simulink model "gm_sampleModel1798_1_sub"  (R2023a)
settings: Solver=VariableStepAuto  StartTime=0.0  StopTime=10.0  RelTol=1e-3
libraries: simulink x2, hdlsllib x1
settings Model: Creator=user1  LastModifiedBy=user1
settings OptimizationCC: BlockReduction=off  ConditionallyExecuteInputs=off
settings DebuggingCC: InheritedTsInSrcMsg=none

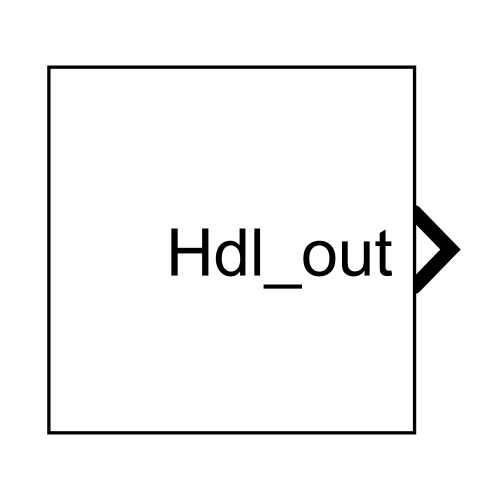
[thumbnail: Simulink's stored preview of the top-level diagram]
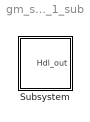
== system gm_sampleModel1798_1_sub ==
  Subsystem : Subsystem

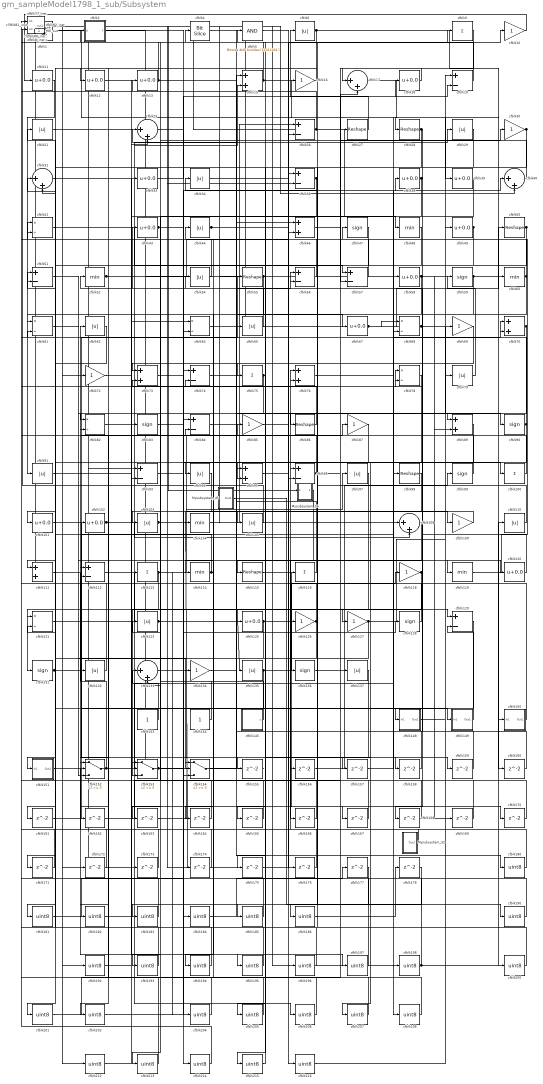
== system gm_sampleModel1798_1_sub/Subsystem ==
  Mysubsystem_32 : Subsystem
  Mysubsystem_36 : Subsystem
  Mysubsystem_45 : Subsystem
  cfblk1 : simulink/Logic and Bit Operations/Extract Bits  bitsToExtract=Upper half  numBits=8  bitIdxRange=[0 7]  outScalingMode=Preserve fixed-point scaling
      settings: LibrarySourceBlock=|
      | hdlsllib/Logic and Bit
      | Operations/Extract Bits
  cfblk{10,16,30,69,72,85,87,109,118,126..127,134} (12 alike) : Gain  OutDataTypeStr=uint8
  cfblk{9,75,100,113,116} (5 alike) : Sum  Inputs=+  OutDataTypeStr=uint8
  cfblk{11..13,18,33,38..39,43,49,58,67,101..102,120,125} (15 alike) : Bias  Bias=0.0  SaturateOnIntegerOverflow=off
  cfblk{6,21,29,34,44,54,62,65,79,91,94,97,103,105,110,123,132,135,137} (19 alike) : Abs  OutDataTypeStr=uint8  SaturateOnIntegerOverflow=off
  cfblk{48,52,60,104,114,119} (6 alike) : MinMax  OutDataTypeStr=uint8
  cfblk106_inst : Subsystem
  cfblk{17,23,31,40,108,133} (6 alike) : Sum  Inputs=|++  OutDataTypeStr=uint8
  cfblk{15,46,70,73,76,89,95,111} (8 alike) : Sum  OutDataTypeStr=uint8
  cfblk{19,26,36,51,56..57,74,84,93,96,112,129} (12 alike) : Sum  Inputs=+-  OutDataTypeStr=uint8
  cfblk{27..28,50,55,86,98,115} (7 alike) : Reshape
  cfblk117_inst : Subsystem
  cfblk{41,61,64,68,78,82,121} (7 alike) : Product  Inputs=*/  OutDataTypeStr=uint8  RndMeth=Zero  SaturateOnIntegerOverflow=on
  cfblk122_inst : Subsystem
  cfblk{47,59,83,90,99,128,131,136} (8 alike) : Signum
  cfblk130_inst : Subsystem
  cfblk143 : Constant  OutDataTypeStr=uint8  SampleTime=-1
  cfblk144 : Constant  OutDataTypeStr=uint8  SampleTime=-1
  cfblk145 : Subsystem  mask(Counter Limited){uplimit=double(7), tsamp=double(-1)}
      mask prompts: uplimit "Simulink:masks:UpperLimit_MP"; tsamp "Simulink:masks:SampleTime_MP"
      mask help: Simulink:masks:CounterLimited_MD
      mask init:
      | nbits = double(8);
      | tsamp = double(-1);
      | uplimit = double(7);
  cfblk148 : Subsystem
  cfblk149 : Subsystem
  cfblk150 : Subsystem
  cfblk151 : Subsystem
  cfblk152 : Switch  OutDataTypeStr=uint8  SaturateOnIntegerOverflow=off  InputSameDT=off
  cfblk153 : Switch  OutDataTypeStr=uint8  SaturateOnIntegerOverflow=off  InputSameDT=off
  cfblk154 : Switch  OutDataTypeStr=uint8  SaturateOnIntegerOverflow=off  InputSameDT=off
  cfblk{155..178} (24 alike) : Delay  SampleTime=1
  cfblk{180..186,190,192..198,200..202,204..208,212..216} (28 alike) : DataTypeConversion  OutDataTypeStr=uint8  SaturateOnIntegerOverflow=off  RndMeth=Floor
  cfblk2 : Subsystem  mask(Detect Rise Positive){vinit=double(0), InputProcessing=Elements as channels (sample based), OutDataTypeStr=uint8}
      mask prompts: vinit "Simulink:masks:InitialCondition_MP"; InputProcessing "Simulink:masks:InputProcessing_MP"; OutDataTypeStr "Simulink:masks:OutputDataType_MP"
      mask help: Simulink:masks:DetectRisePositive_MD
      mask init:
      | InputProcessing = 'Elements as channels (sample based)';
      | OutDataTypeStr = 'uint8';
      | vinit = double(0);
      mask TypeOptions InputProcessing: Simulink:masks:ColumnsAsChannelsFrameBased | Simulink:masks:ElementsAsChannelsSampleBased
      mask TypeOptions OutDataTypeStr: Simulink:masks:uint8 | Simulink:masks:boolean
      mask Display: fprintf('U > 0\n&  NOT\nU/z > 0')
  cfblk20_inst : Subsystem
  cfblk32_inst : Subsystem
  cfblk35_inst : Subsystem
  cfblk4 : hdlsllib/Logic and Bit Operations/Bit Slice  lidx=7  ridx=0
  cfblk45_inst : Subsystem
  cfblk5 : simulink/Logic and Bit Operations/Bitwise Operator  logicop=AND  UseBitMask=on  BitMask=bin2dec('11011001')  BitMaskRealWorld=Stored Integer
      settings: LibrarySourceBlock=|
      | hdlsllib/Logic and Bit
      | Operations/Bitwise
      | Operator
  cfblk53_inst : Subsystem
  cfblk63_inst : Subsystem
  cfblk77_inst : Subsystem
  cfblk80_inst : Subsystem
  cfblk81_inst : Subsystem
  cfblk8_inst : Subsystem
  cfblk92_inst : Subsystem
  Hdl_out : Outport  OutDataTypeStr=uint8  SampleTime=1
  wires:
  Mysubsystem_32/1(Out1) -> cfblk76/1
  Mysubsystem_36/1(Out1) -> cfblk166/1
  Mysubsystem_45/1(Out1) -> cfblk190/1
  cfblk1/1 -> cfblk28/1
  cfblk10/1 -> cfblk11/1
  cfblk100/1 -> cfblk34/1
  cfblk101/1 -> cfblk158/1
  cfblk102/1 -> cfblk29/1, cfblk108/2
  cfblk103/1 -> cfblk174/1, cfblk109/1
  cfblk104/1 -> cfblk26/1
  cfblk105/1 -> cfblk81_inst/2(in2)
  cfblk106_inst/1(out1) -> cfblk36/2, cfblk111/2
  cfblk108/1 -> cfblk115/1
  cfblk109/1 -> cfblk105/1
  cfblk11/1 -> cfblk91/1
  cfblk110/1 -> cfblk2/1(U)
  cfblk111/1 -> cfblk197/1
  cfblk112/1 -> cfblk206/1
  cfblk113/1 -> cfblk97/1, cfblk204/1, cfblk153/3, cfblk85/1
  cfblk114/1 -> cfblk51/1, cfblk194/1
  cfblk115/1 -> cfblk159/1
  cfblk116/1 -> cfblk23/1
  cfblk117_inst/1(out1) -> cfblk108/1, cfblk172/1
  cfblk118/1 -> cfblk207/1, cfblk131/1
  cfblk119/1 -> cfblk47/1
  cfblk12/1 -> cfblk23/2
  cfblk120/1 -> cfblk52/1
  cfblk121/1 -> cfblk15/2
  cfblk122_inst/1(out1) -> cfblk192/1
  cfblk123/1 -> cfblk213/1, cfblk135/1
  cfblk125/1 -> cfblk167/1, cfblk151/1(In1)
  cfblk126/1 -> cfblk96/1, cfblk154/2
  cfblk127/1 -> cfblk49/1, cfblk171/1
  cfblk128/1 -> cfblk62/1
  cfblk129/1 -> cfblk181/1
  cfblk13/1 -> cfblk77_inst/1(in1), cfblk119/1
  cfblk130_inst/1(out1) -> cfblk93/1, cfblk176/1
  cfblk131/1 -> cfblk84/2, cfblk149/1(In1)
  cfblk132/1 -> cfblk45_inst/2(in2)
  cfblk133/1 -> cfblk155/1
  cfblk134/1 -> cfblk46/1
  cfblk135/1 -> cfblk154/1, cfblk118/1
  cfblk136/1 -> cfblk99/1
  cfblk137/1 -> cfblk205/1
  cfblk143/1 -> cfblk133/1
  cfblk144/1 -> cfblk117_inst/2(in2)
  cfblk145/1(y) -> cfblk41/1
  cfblk148/1(Out1) -> cfblk70/1
  cfblk149/1(Out1) -> cfblk129/2
  cfblk15/1 -> cfblk4/1, cfblk68/2, cfblk150/1(In1)
  cfblk150/1(Out1) -> cfblk56/1
  cfblk151/1(Out1) -> cfblk55/1
  cfblk152/1 -> cfblk98/1, cfblk102/1
  cfblk153/1 -> cfblk128/1, cfblk123/1
  cfblk154/1 -> cfblk56/2
  cfblk155/1 -> cfblk1/1
  cfblk156/1 -> cfblk19/1
  cfblk157/1 -> cfblk40/1
  cfblk158/1 -> cfblk15/1
  cfblk159/1 -> cfblk78/1
  cfblk16/1 -> cfblk12/1
  cfblk160/1 -> cfblk36/1
  cfblk161/1 -> cfblk70/2
  cfblk162/1 -> cfblk46/2
  cfblk163/1 -> cfblk17/2
  cfblk164/1 -> cfblk63_inst/2(in2)
  cfblk165/1 -> cfblk32_inst/2(in2)
  cfblk166/1 -> cfblk61/2
  cfblk167/1 -> cfblk51/2
  cfblk168/1 -> cfblk121/2
  cfblk169/1 -> cfblk73/2
  cfblk17/1 -> cfblk39/1
  cfblk170/1 -> cfblk153/1
  cfblk171/1 -> cfblk130_inst/1(in1)
  cfblk172/1 -> cfblk81_inst/1(in1)
  cfblk173/1 -> cfblk82/2
  cfblk174/1 -> cfblk152/2
  cfblk175/1 -> cfblk26/2
  cfblk176/1 -> cfblk106_inst/2(in2)
  cfblk177/1 -> cfblk183/1
  cfblk178/1 -> cfblk185/1
  cfblk18/1 -> cfblk17/1
  cfblk180/1 -> cfblk35_inst/2(in2)
  cfblk181/1 -> cfblk74/1
  cfblk182/1 -> cfblk74/2
  cfblk183/1 -> cfblk35_inst/1(in1)
  cfblk184/1 -> cfblk177/1
  cfblk185/1 -> cfblk8_inst/1(in1)
  cfblk186/1 -> cfblk178/1
  cfblk19/1 -> cfblk106_inst/1(in1)
  cfblk190/1 -> cfblk8_inst/2(in2)
  cfblk192/1 -> cfblk33/1
  cfblk193/1 -> cfblk122_inst/1(in1)
  cfblk194/1 -> cfblk122_inst/2(in2)
  cfblk195/1 -> cfblk20_inst/2(in2)
  cfblk196/1 -> cfblk31/1
  cfblk197/1 -> cfblk31/2
  cfblk198/1 -> cfblk20_inst/1(in1), cfblk110/1
  cfblk2/1(Y) -> cfblk184/1
  cfblk20_inst/1(out1) -> cfblk58/1
  cfblk200/1 -> cfblk76/2
  cfblk201/1 -> cfblk137/1
  cfblk202/1 -> cfblk87/1
  cfblk204/1 -> cfblk80_inst/1(in1)
  cfblk205/1 -> cfblk80_inst/2(in2)
  cfblk206/1 -> cfblk44/1
  cfblk207/1 -> cfblk112/1
  cfblk208/1 -> cfblk112/2
  cfblk21/1 -> cfblk48/1
  cfblk212/1 -> cfblk64/1
  cfblk213/1 -> cfblk92_inst/1(in1)
  cfblk214/1 -> cfblk92_inst/2(in2)
  cfblk215/1 -> cfblk5/1
  cfblk216/1 -> cfblk79/1
  cfblk23/1 -> cfblk84/1
  cfblk26/1 -> cfblk208/1, cfblk130_inst/2(in2)
  cfblk27/1 -> cfblk6/1
  cfblk28/1 -> cfblk182/1, cfblk148/1(In1)
  cfblk29/1 -> cfblk101/1
  cfblk30/1 -> cfblk136/1, cfblk125/1
  cfblk31/1 -> cfblk195/1
  cfblk32_inst/1(out1) -> cfblk40/2
  cfblk33/1 -> cfblk18/1
  cfblk34/1 -> cfblk196/1
  cfblk35_inst/1(out1) -> cfblk200/1
  cfblk36/1 -> cfblk86/1, cfblk133/2
  cfblk38/1 -> cfblk95/2, cfblk75/1
  cfblk39/1 -> cfblk96/2
  cfblk4/1 -> cfblk67/1
  cfblk40/1 -> cfblk13/1
  cfblk41/1 -> cfblk57/1
  cfblk43/1 -> cfblk214/1, cfblk100/1
  cfblk44/1 -> cfblk65/1, cfblk10/1
  cfblk45_inst/1(out1) -> cfblk27/1
  cfblk46/1 -> cfblk19/2
  cfblk47/1 -> cfblk61/1
  cfblk48/1 -> cfblk64/2
  cfblk49/1 -> cfblk103/1, cfblk175/1
  cfblk5/1 -> cfblk216/1
  cfblk50/1 -> cfblk93/2, cfblk41/2
  cfblk51/1 -> cfblk134/1
  cfblk52/1 -> cfblk153/2, cfblk16/1
  cfblk53_inst/1(out1) -> cfblk60/1
  cfblk54/1 -> cfblk53_inst/1(in1)
  cfblk55/1 -> cfblk202/1, cfblk165/1, cfblk164/1, Hdl_out/1
  cfblk56/1 -> cfblk63_inst/1(in1)
  cfblk57/1 -> cfblk45_inst/1(in1)
  cfblk58/1 -> cfblk94/1, cfblk169/1, cfblk168/1
  cfblk59/1 -> cfblk152/1, cfblk111/1
  cfblk6/1 -> cfblk162/1, cfblk161/1, cfblk160/1
  cfblk60/1 -> cfblk21/1, cfblk132/1, cfblk163/1
  cfblk61/1 -> cfblk120/1
  cfblk62/1 -> cfblk121/1
  cfblk63_inst/1(out1) -> cfblk69/1
  cfblk64/1 -> cfblk89/1
  cfblk65/1 -> cfblk43/1
  cfblk67/1 -> cfblk50/1, cfblk68/1
  cfblk68/1 -> cfblk90/1, cfblk89/2
  cfblk69/1 -> cfblk73/1
  cfblk70/1 -> cfblk152/3, cfblk114/1
  cfblk72/1 -> cfblk126/1
  cfblk73/1 -> cfblk38/1
  cfblk74/1 -> cfblk180/1
  cfblk75/1 -> cfblk95/1, cfblk82/1
  cfblk76/1 -> cfblk198/1
  cfblk77_inst/1(out1) -> cfblk72/1
  cfblk78/1 -> cfblk215/1
  cfblk79/1 -> cfblk59/1
  cfblk8_inst/1(out1) -> cfblk113/1
  cfblk80_inst/1(out1) -> Mysubsystem_36/1(In1)
  cfblk81_inst/1(out1) -> cfblk117_inst/1(in1), cfblk173/1
  cfblk82/1 -> cfblk83/1
  cfblk83/1 -> cfblk78/2
  cfblk84/1 -> cfblk156/1
  cfblk85/1 -> cfblk9/1
  cfblk86/1 -> cfblk32_inst/1(in1)
  cfblk87/1 -> cfblk201/1
  cfblk89/1 -> cfblk116/1
  cfblk9/1 -> cfblk57/2
  cfblk90/1 -> cfblk77_inst/2(in2), cfblk154/3, cfblk157/1
  cfblk91/1 -> cfblk170/1
  cfblk92_inst/1(out1) -> cfblk212/1
  cfblk93/1 -> cfblk127/1
  cfblk94/1 -> cfblk193/1
  cfblk95/1 -> cfblk129/1
  cfblk96/1 -> cfblk53_inst/2(in2), cfblk30/1
  cfblk97/1 -> cfblk186/1
  cfblk98/1 -> cfblk104/1
  cfblk99/1 -> cfblk54/1

== system gm_sampleModel1798_1_sub/Subsystem/Mysubsystem_32 ==
  cfblk147 : Subsystem  mask(Counter Free-Running){NumBits=double(16), tsamp=double(-1)}
      mask prompts: NumBits "Simulink:masks:NumberOfBits_MP"; tsamp "Simulink:masks:SampleTime_MP"
      mask help: Simulink:masks:CounterFreeRunning_MD
  cfblk199 : DataTypeConversion  OutDataTypeStr=uint8  SaturateOnIntegerOverflow=off  RndMeth=Floor
  Out1 : Outport  SampleTime=1
  wires:
  cfblk147/1(y) -> cfblk199/1
  cfblk199/1 -> Out1/1

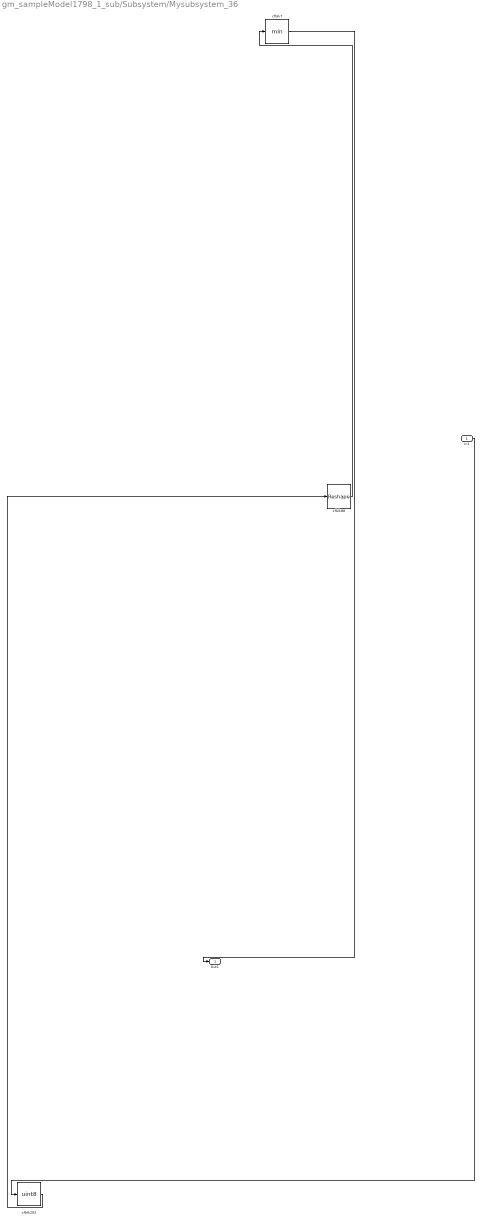
== system gm_sampleModel1798_1_sub/Subsystem/Mysubsystem_36 ==
  In1 : Inport  OutDataTypeStr=uint8  PortDimensions=1  SampleTime=1
  cfblk203 : DataTypeConversion  OutDataTypeStr=uint8  SaturateOnIntegerOverflow=off  RndMeth=Floor
  cfblk7 : MinMax
  cfblk88 : Reshape
  Out1 : Outport  SampleTime=1
  wires:
  In1/1 -> cfblk203/1
  cfblk203/1 -> cfblk88/1
  cfblk7/1 -> Out1/1
  cfblk88/1 -> cfblk7/1

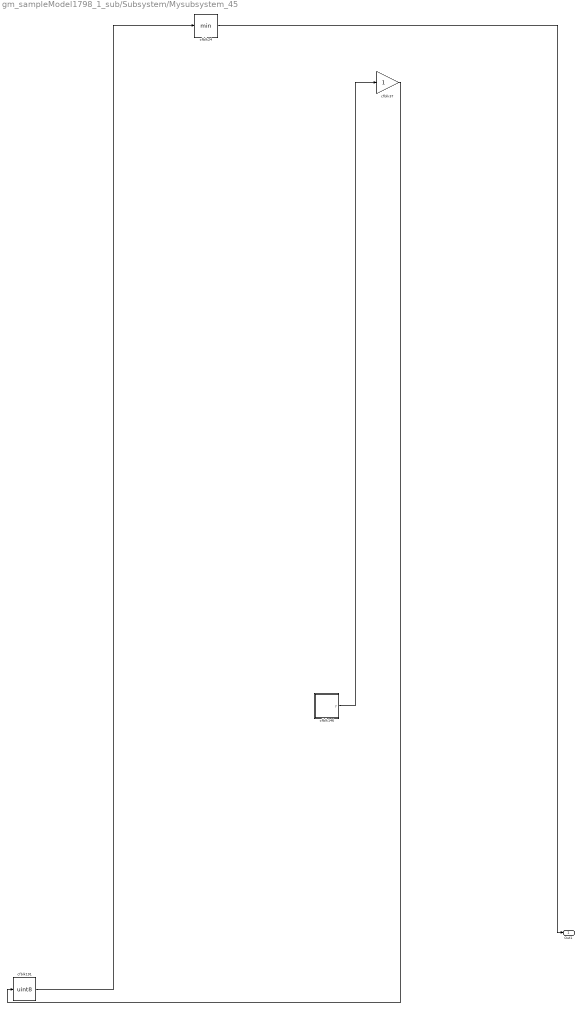
== system gm_sampleModel1798_1_sub/Subsystem/Mysubsystem_45 ==
  cfblk146 : Subsystem  mask(Counter Limited){uplimit=double(7), tsamp=double(-1)}
      mask prompts: uplimit "Simulink:masks:UpperLimit_MP"; tsamp "Simulink:masks:SampleTime_MP"
      mask help: Simulink:masks:CounterLimited_MD
      mask init:
      | nbits = double(8);
      | tsamp = double(-1);
      | uplimit = double(7);
  cfblk191 : DataTypeConversion  OutDataTypeStr=uint8  SaturateOnIntegerOverflow=off  RndMeth=Floor
  cfblk24 : MinMax
  cfblk37 : Gain
  Out1 : Outport  SampleTime=1
  wires:
  cfblk146/1(y) -> cfblk37/1
  cfblk191/1 -> cfblk24/1
  cfblk24/1 -> Out1/1
  cfblk37/1 -> cfblk191/1

== system gm_sampleModel1798_1_sub/Subsystem/cfblk106_inst ==
  in1 : Inport  OutDataTypeStr=uint8  SampleTime=1
  in2 : Inport  Port=2  OutDataTypeStr=uint8  SampleTime=1
  mul_cfblk106_dotp_mulcomp : Product  Inputs=**  OutDataTypeStr=uint8  SampleTime=1
  out1 : Outport  OutDataTypeStr=uint8  SampleTime=1
  wires:
  in1/1 -> mul_cfblk106_dotp_mulcomp/1
  in2/1 -> mul_cfblk106_dotp_mulcomp/2
  mul_cfblk106_dotp_mulcomp/1 -> out1/1

== system gm_sampleModel1798_1_sub/Subsystem/cfblk117_inst ==
  in1 : Inport  OutDataTypeStr=uint8  SampleTime=1
  in2 : Inport  Port=2  OutDataTypeStr=uint8  SampleTime=1
  mul_cfblk117_dotp_mulcomp : Product  Inputs=**  OutDataTypeStr=uint8  SampleTime=1
  out1 : Outport  OutDataTypeStr=uint8  SampleTime=1
  wires:
  in1/1 -> mul_cfblk117_dotp_mulcomp/1
  in2/1 -> mul_cfblk117_dotp_mulcomp/2
  mul_cfblk117_dotp_mulcomp/1 -> out1/1

== system gm_sampleModel1798_1_sub/Subsystem/cfblk122_inst ==
  in1 : Inport  OutDataTypeStr=uint8  SampleTime=1
  in2 : Inport  Port=2  OutDataTypeStr=uint8  SampleTime=1
  mul_cfblk122_dotp_mulcomp : Product  Inputs=**  OutDataTypeStr=uint8  SampleTime=1
  out1 : Outport  OutDataTypeStr=uint8  SampleTime=1
  wires:
  in1/1 -> mul_cfblk122_dotp_mulcomp/1
  in2/1 -> mul_cfblk122_dotp_mulcomp/2
  mul_cfblk122_dotp_mulcomp/1 -> out1/1

== system gm_sampleModel1798_1_sub/Subsystem/cfblk130_inst ==
  in1 : Inport  OutDataTypeStr=uint8  SampleTime=1
  in2 : Inport  Port=2  OutDataTypeStr=uint8  SampleTime=1
  mul_cfblk130_dotp_mulcomp : Product  Inputs=**  OutDataTypeStr=uint8  SampleTime=1
  out1 : Outport  OutDataTypeStr=uint8  SampleTime=1
  wires:
  in1/1 -> mul_cfblk130_dotp_mulcomp/1
  in2/1 -> mul_cfblk130_dotp_mulcomp/2
  mul_cfblk130_dotp_mulcomp/1 -> out1/1

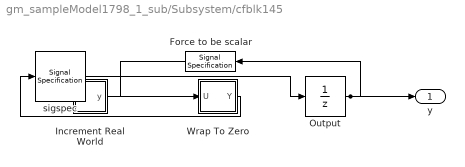
== system gm_sampleModel1798_1_sub/Subsystem/cfblk145 ==
  Force to be scalar : SignalSpecification  DisableCoverage=on  Dimensions=1
  Increment Real World : Subsystem  mask(Real World Value Increment){}
      mask help: Simulink:masks:RealWorldValueIncrement_MD
      mask Display: disp('V++')
  Output : UnitDelay  InitialCondition=0.0  SampleTime=tsamp  HasFrameUpgradeWarning=on
  Wrap To Zero : Subsystem  mask(Wrap To Zero){Threshold=double(7)}
      mask prompts: Threshold "Simulink:masks:Threshold_MP"
      mask help: Simulink:masks:WrapToZero_MD
  sigspec : SignalSpecification  OutDataTypeStr=uint8  Dimensions=1
  y : Outport  SampleTime=1
  wires:
  Force to be scalar/1 -> Increment Real World/1(u)
  Increment Real World/1(y) -> Wrap To Zero/1(U)
  Output/1 -> Force to be scalar/1, y/1
  Wrap To Zero/1(Y) -> sigspec/1
  sigspec/1 -> Output/1

== system gm_sampleModel1798_1_sub/Subsystem/cfblk148 ==
  In1 : Inport  OutDataTypeStr=fixdt(0, 4, -4)  PortDimensions=1  SampleTime=1
  Out1 : Outport  SampleTime=1
  wires:
  In1/1 -> Out1/1

== system gm_sampleModel1798_1_sub/Subsystem/cfblk149 ==
  In1 : Inport  OutDataTypeStr=uint8  PortDimensions=1  SampleTime=1
  Out1 : Outport  SampleTime=1
  wires:
  In1/1 -> Out1/1

== system gm_sampleModel1798_1_sub/Subsystem/cfblk150 ==
  In1 : Inport  OutDataTypeStr=uint8  PortDimensions=1  SampleTime=1
  Out1 : Outport  SampleTime=1
  wires:
  In1/1 -> Out1/1

== system gm_sampleModel1798_1_sub/Subsystem/cfblk151 ==
  In1 : Inport  OutDataTypeStr=uint8  PortDimensions=1  SampleTime=1
  Out1 : Outport  SampleTime=1
  wires:
  In1/1 -> Out1/1

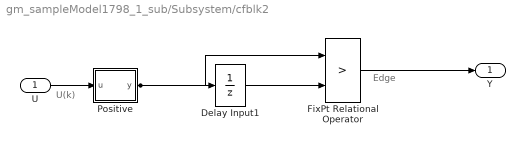
== system gm_sampleModel1798_1_sub/Subsystem/cfblk2 ==
  note: U(k)
  note: Edge
  U : Inport  OutDataTypeStr=uint8  SampleTime=1
  Delay Input1 : UnitDelay  Description=Store in Global RAM  DisableCoverage=on  InitialCondition=vinit  SampleTime=-1  HasFrameUpgradeWarning=on
  FixPt Relational Operator : RelationalOperator  Operator=>  OutDataTypeStr=fixdt(0, 8)  ZeroCross=off  InputSameDT=off
  Positive : Subsystem  mask(Compare To Zero){relop=>, OutDataTypeStr=boolean, ZeroCross=off}
      mask prompts: relop "Simulink:masks:Operator_MP"; OutDataTypeStr "Simulink:masks:OutputDataType_MP"; ZeroCross "Simulink:masks:EnableZerocrossingDetection_MP"
      mask help: Simulink:masks:CompareToZero_MD
      mask init:
      | OutDataTypeStr = 'boolean';
      | ZeroCross = 'off';
      | blkName = 'sampleModel1798_1_sub/Subsystem/cfblk2/Positive';
      | relop = '>';
      | setValue = 'boolean';
      mask TypeOptions relop: == | ~= | < | <= | >= | >
      mask TypeOptions OutDataTypeStr: Simulink:masks:uint8 | Simulink:masks:boolean
      mask Callback ZeroCross: sl('zeroCrossEnable', gcbh);
      mask Display: disp([relop,' 0'])
  Y : Outport  SampleTime=1
  wires:
  U/1 -> Positive/1(u)
  Delay Input1/1 -> FixPt Relational Operator/2
  FixPt Relational Operator/1 -> Y/1
  Positive/1(y) -> FixPt Relational Operator/1, Delay Input1/1

== system gm_sampleModel1798_1_sub/Subsystem/cfblk20_inst ==
  in1 : Inport  OutDataTypeStr=uint8  SampleTime=1
  in2 : Inport  Port=2  OutDataTypeStr=uint8  SampleTime=1
  mul_cfblk20_dotp_mulcomp : Product  Inputs=**  OutDataTypeStr=uint8  SampleTime=1
  out1 : Outport  OutDataTypeStr=uint8  SampleTime=1
  wires:
  in1/1 -> mul_cfblk20_dotp_mulcomp/1
  in2/1 -> mul_cfblk20_dotp_mulcomp/2
  mul_cfblk20_dotp_mulcomp/1 -> out1/1

== system gm_sampleModel1798_1_sub/Subsystem/cfblk32_inst ==
  in1 : Inport  OutDataTypeStr=uint8  SampleTime=1
  in2 : Inport  Port=2  OutDataTypeStr=uint8  SampleTime=1
  mul_cfblk32_dotp_mulcomp : Product  Inputs=**  OutDataTypeStr=uint8  SampleTime=1
  out1 : Outport  OutDataTypeStr=uint8  SampleTime=1
  wires:
  in1/1 -> mul_cfblk32_dotp_mulcomp/1
  in2/1 -> mul_cfblk32_dotp_mulcomp/2
  mul_cfblk32_dotp_mulcomp/1 -> out1/1

== system gm_sampleModel1798_1_sub/Subsystem/cfblk35_inst ==
  in1 : Inport  OutDataTypeStr=uint8  SampleTime=1
  in2 : Inport  Port=2  OutDataTypeStr=uint8  SampleTime=1
  mul_cfblk35_dotp_mulcomp : Product  Inputs=**  OutDataTypeStr=uint8  SampleTime=1
  out1 : Outport  OutDataTypeStr=uint8  SampleTime=1
  wires:
  in1/1 -> mul_cfblk35_dotp_mulcomp/1
  in2/1 -> mul_cfblk35_dotp_mulcomp/2
  mul_cfblk35_dotp_mulcomp/1 -> out1/1

== system gm_sampleModel1798_1_sub/Subsystem/cfblk45_inst ==
  in1 : Inport  OutDataTypeStr=uint8  SampleTime=1
  in2 : Inport  Port=2  OutDataTypeStr=uint8  SampleTime=1
  mul_cfblk45_dotp_mulcomp : Product  Inputs=**  OutDataTypeStr=uint8  SampleTime=1
  out1 : Outport  OutDataTypeStr=uint8  SampleTime=1
  wires:
  in1/1 -> mul_cfblk45_dotp_mulcomp/1
  in2/1 -> mul_cfblk45_dotp_mulcomp/2
  mul_cfblk45_dotp_mulcomp/1 -> out1/1

== system gm_sampleModel1798_1_sub/Subsystem/cfblk53_inst ==
  in1 : Inport  OutDataTypeStr=uint8  SampleTime=1
  in2 : Inport  Port=2  OutDataTypeStr=uint8  SampleTime=1
  mul_cfblk53_dotp_mulcomp : Product  Inputs=**  OutDataTypeStr=uint8  SampleTime=1
  out1 : Outport  OutDataTypeStr=uint8  SampleTime=1
  wires:
  in1/1 -> mul_cfblk53_dotp_mulcomp/1
  in2/1 -> mul_cfblk53_dotp_mulcomp/2
  mul_cfblk53_dotp_mulcomp/1 -> out1/1

== system gm_sampleModel1798_1_sub/Subsystem/cfblk63_inst ==
  in1 : Inport  OutDataTypeStr=uint8  SampleTime=1
  in2 : Inport  Port=2  OutDataTypeStr=uint8  SampleTime=1
  mul_cfblk63_dotp_mulcomp : Product  Inputs=**  OutDataTypeStr=uint8  SampleTime=1
  out1 : Outport  OutDataTypeStr=uint8  SampleTime=1
  wires:
  in1/1 -> mul_cfblk63_dotp_mulcomp/1
  in2/1 -> mul_cfblk63_dotp_mulcomp/2
  mul_cfblk63_dotp_mulcomp/1 -> out1/1

== system gm_sampleModel1798_1_sub/Subsystem/cfblk77_inst ==
  in1 : Inport  OutDataTypeStr=uint8  SampleTime=1
  in2 : Inport  Port=2  OutDataTypeStr=uint8  SampleTime=1
  mul_cfblk77_dotp_mulcomp : Product  Inputs=**  OutDataTypeStr=uint8  SampleTime=1
  out1 : Outport  OutDataTypeStr=uint8  SampleTime=1
  wires:
  in1/1 -> mul_cfblk77_dotp_mulcomp/1
  in2/1 -> mul_cfblk77_dotp_mulcomp/2
  mul_cfblk77_dotp_mulcomp/1 -> out1/1

== system gm_sampleModel1798_1_sub/Subsystem/cfblk80_inst ==
  in1 : Inport  OutDataTypeStr=uint8  SampleTime=1
  in2 : Inport  Port=2  OutDataTypeStr=uint8  SampleTime=1
  mul_cfblk80_dotp_mulcomp : Product  Inputs=**  OutDataTypeStr=uint8  SampleTime=1
  out1 : Outport  OutDataTypeStr=uint8  SampleTime=1
  wires:
  in1/1 -> mul_cfblk80_dotp_mulcomp/1
  in2/1 -> mul_cfblk80_dotp_mulcomp/2
  mul_cfblk80_dotp_mulcomp/1 -> out1/1

== system gm_sampleModel1798_1_sub/Subsystem/cfblk81_inst ==
  in1 : Inport  OutDataTypeStr=uint8  SampleTime=1
  in2 : Inport  Port=2  OutDataTypeStr=uint8  SampleTime=1
  mul_cfblk81_dotp_mulcomp : Product  Inputs=**  OutDataTypeStr=uint8  SampleTime=1
  out1 : Outport  OutDataTypeStr=uint8  SampleTime=1
  wires:
  in1/1 -> mul_cfblk81_dotp_mulcomp/1
  in2/1 -> mul_cfblk81_dotp_mulcomp/2
  mul_cfblk81_dotp_mulcomp/1 -> out1/1

== system gm_sampleModel1798_1_sub/Subsystem/cfblk8_inst ==
  in1 : Inport  OutDataTypeStr=uint8  SampleTime=1
  in2 : Inport  Port=2  OutDataTypeStr=uint8  SampleTime=1
  mul_cfblk8_dotp_mulcomp : Product  Inputs=**  OutDataTypeStr=uint8  SampleTime=1
  out1 : Outport  OutDataTypeStr=uint8  SampleTime=1
  wires:
  in1/1 -> mul_cfblk8_dotp_mulcomp/1
  in2/1 -> mul_cfblk8_dotp_mulcomp/2
  mul_cfblk8_dotp_mulcomp/1 -> out1/1

== system gm_sampleModel1798_1_sub/Subsystem/cfblk92_inst ==
  in1 : Inport  OutDataTypeStr=uint8  SampleTime=1
  in2 : Inport  Port=2  OutDataTypeStr=uint8  SampleTime=1
  mul_cfblk92_dotp_mulcomp : Product  Inputs=**  OutDataTypeStr=uint8  SampleTime=1
  out1 : Outport  OutDataTypeStr=uint8  SampleTime=1
  wires:
  in1/1 -> mul_cfblk92_dotp_mulcomp/1
  in2/1 -> mul_cfblk92_dotp_mulcomp/2
  mul_cfblk92_dotp_mulcomp/1 -> out1/1

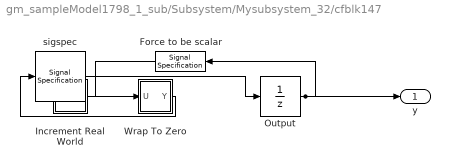
== system gm_sampleModel1798_1_sub/Subsystem/Mysubsystem_32/cfblk147 ==
  Force to be scalar : SignalSpecification  DisableCoverage=on  Dimensions=1
  Increment Real World : Subsystem  mask(Real World Value Increment){}
      mask help: Simulink:masks:RealWorldValueIncrement_MD
      mask Display: disp('V++')
  Output : UnitDelay  InitialCondition=0.0  SampleTime=tsamp  HasFrameUpgradeWarning=on
  Wrap To Zero : Subsystem  mask(Wrap To Zero){Threshold=double(65535)}
      mask prompts: Threshold "Simulink:masks:Threshold_MP"
      mask help: Simulink:masks:WrapToZero_MD
  sigspec : SignalSpecification  OutDataTypeStr=uint16  Dimensions=1
  y : Outport  SampleTime=1
  wires:
  Force to be scalar/1 -> Increment Real World/1(u)
  Increment Real World/1(y) -> Wrap To Zero/1(U)
  Output/1 -> Force to be scalar/1, y/1
  Wrap To Zero/1(Y) -> sigspec/1
  sigspec/1 -> Output/1

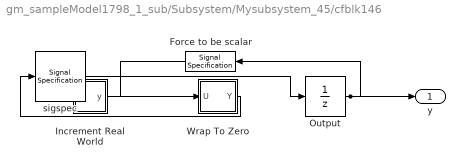
== system gm_sampleModel1798_1_sub/Subsystem/Mysubsystem_45/cfblk146 ==
  Force to be scalar : SignalSpecification  DisableCoverage=on  Dimensions=1
  Increment Real World : Subsystem  mask(Real World Value Increment){}
      mask help: Simulink:masks:RealWorldValueIncrement_MD
      mask Display: disp('V++')
  Output : UnitDelay  InitialCondition=0.0  SampleTime=tsamp  HasFrameUpgradeWarning=on
  Wrap To Zero : Subsystem  mask(Wrap To Zero){Threshold=double(7)}
      mask prompts: Threshold "Simulink:masks:Threshold_MP"
      mask help: Simulink:masks:WrapToZero_MD
  sigspec : SignalSpecification  OutDataTypeStr=uint8  Dimensions=1
  y : Outport  SampleTime=1
  wires:
  Force to be scalar/1 -> Increment Real World/1(u)
  Increment Real World/1(y) -> Wrap To Zero/1(U)
  Output/1 -> Force to be scalar/1, y/1
  Wrap To Zero/1(Y) -> sigspec/1
  sigspec/1 -> Output/1

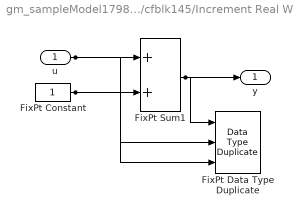
== system gm_sampleModel1798_1_sub/Subsystem/cfblk145/Increment Real World ==
  u : Inport  OutDataTypeStr=uint8  SampleTime=1
  FixPt Constant : Constant  DisableCoverage=on  OutDataTypeStr=Inherit: Inherit via back propagation  SampleTime=-1
  FixPt Data Type Duplicate : DataTypeDuplicate  DisableCoverage=on  NumInputPorts=3
  FixPt Sum1 : Sum  InputSameDT=on  OutDataTypeStr=Inherit: Inherit via back propagation  LockScale=on
  y : Outport  SampleTime=1
  wires:
  u/1 -> FixPt Sum1/1, FixPt Data Type Duplicate/2
  FixPt Constant/1 -> FixPt Sum1/2, FixPt Data Type Duplicate/3
  FixPt Sum1/1 -> FixPt Data Type Duplicate/1, y/1

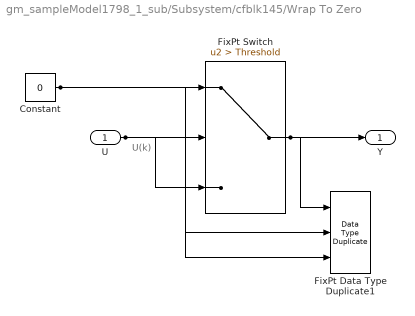
== system gm_sampleModel1798_1_sub/Subsystem/cfblk145/Wrap To Zero ==
  note: U(k)
  U : Inport  OutDataTypeStr=uint8  SampleTime=1
  Constant : Constant  DisableCoverage=on  Value=0  OutDataTypeStr=Inherit: Inherit via back propagation  SampleTime=-1
  FixPt Data Type Duplicate1 : DataTypeDuplicate  DisableCoverage=on  NumInputPorts=3
  FixPt Switch : Switch  Criteria=u2 > Threshold  Threshold=Threshold  OutDataTypeStr=Inherit: Inherit via back propagation  ZeroCross=off  SaturateOnIntegerOverflow=off  InputSameDT=off
  Y : Outport  SampleTime=1
  wires:
  U/1 -> FixPt Switch/3, FixPt Switch/2, FixPt Data Type Duplicate1/2
  Constant/1 -> FixPt Switch/1, FixPt Data Type Duplicate1/3
  FixPt Switch/1 -> FixPt Data Type Duplicate1/1, Y/1

== system gm_sampleModel1798_1_sub/Subsystem/cfblk2/Positive ==
  u : Inport  OutDataTypeStr=uint8  SampleTime=1
  Compare : RelationalOperator  Operator=>  OutDataTypeStr=boolean  ZeroCross=off
  Constant : Constant  DisableCoverage=on  Value=0  OutDataTypeStr=Inherit: Inherit via back propagation  SampleTime=-1  PreserveConstantTs=on
  y : Outport  SampleTime=1
  wires:
  u/1 -> Compare/1
  Compare/1 -> y/1
  Constant/1 -> Compare/2

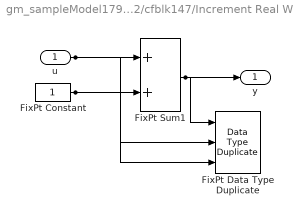
== system gm_sampleModel1798_1_sub/Subsystem/Mysubsystem_32/cfblk147/Increment Real World ==
  u : Inport  OutDataTypeStr=uint16  SampleTime=1
  FixPt Constant : Constant  DisableCoverage=on  OutDataTypeStr=Inherit: Inherit via back propagation  SampleTime=-1
  FixPt Data Type Duplicate : DataTypeDuplicate  DisableCoverage=on  NumInputPorts=3
  FixPt Sum1 : Sum  InputSameDT=on  OutDataTypeStr=Inherit: Inherit via back propagation  LockScale=on
  y : Outport  SampleTime=1
  wires:
  u/1 -> FixPt Sum1/1, FixPt Data Type Duplicate/2
  FixPt Constant/1 -> FixPt Sum1/2, FixPt Data Type Duplicate/3
  FixPt Sum1/1 -> FixPt Data Type Duplicate/1, y/1

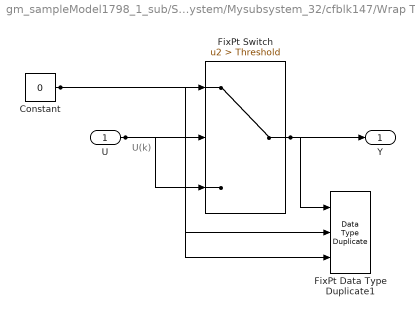
== system gm_sampleModel1798_1_sub/Subsystem/Mysubsystem_32/cfblk147/Wrap To Zero ==
  note: U(k)
  U : Inport  OutDataTypeStr=uint16  SampleTime=1
  Constant : Constant  DisableCoverage=on  Value=0  OutDataTypeStr=Inherit: Inherit via back propagation  SampleTime=-1
  FixPt Data Type Duplicate1 : DataTypeDuplicate  DisableCoverage=on  NumInputPorts=3
  FixPt Switch : Switch  Criteria=u2 > Threshold  Threshold=Threshold  OutDataTypeStr=Inherit: Inherit via back propagation  ZeroCross=off  SaturateOnIntegerOverflow=off  InputSameDT=off
  Y : Outport  SampleTime=1
  wires:
  U/1 -> FixPt Switch/3, FixPt Switch/2, FixPt Data Type Duplicate1/2
  Constant/1 -> FixPt Switch/1, FixPt Data Type Duplicate1/3
  FixPt Switch/1 -> FixPt Data Type Duplicate1/1, Y/1

== system gm_sampleModel1798_1_sub/Subsystem/Mysubsystem_45/cfblk146/Increment Real World ==
  u : Inport  OutDataTypeStr=uint8  SampleTime=1
  FixPt Constant : Constant  DisableCoverage=on  OutDataTypeStr=Inherit: Inherit via back propagation  SampleTime=-1
  FixPt Data Type Duplicate : DataTypeDuplicate  DisableCoverage=on  NumInputPorts=3
  FixPt Sum1 : Sum  InputSameDT=on  OutDataTypeStr=Inherit: Inherit via back propagation  LockScale=on
  y : Outport  SampleTime=1
  wires:
  u/1 -> FixPt Sum1/1, FixPt Data Type Duplicate/2
  FixPt Constant/1 -> FixPt Sum1/2, FixPt Data Type Duplicate/3
  FixPt Sum1/1 -> FixPt Data Type Duplicate/1, y/1

== system gm_sampleModel1798_1_sub/Subsystem/Mysubsystem_45/cfblk146/Wrap To Zero ==
  note: U(k)
  U : Inport  OutDataTypeStr=uint8  SampleTime=1
  Constant : Constant  DisableCoverage=on  Value=0  OutDataTypeStr=Inherit: Inherit via back propagation  SampleTime=-1
  FixPt Data Type Duplicate1 : DataTypeDuplicate  DisableCoverage=on  NumInputPorts=3
  FixPt Switch : Switch  Criteria=u2 > Threshold  Threshold=Threshold  OutDataTypeStr=Inherit: Inherit via back propagation  ZeroCross=off  SaturateOnIntegerOverflow=off  InputSameDT=off
  Y : Outport  SampleTime=1
  wires:
  U/1 -> FixPt Switch/3, FixPt Switch/2, FixPt Data Type Duplicate1/2
  Constant/1 -> FixPt Switch/1, FixPt Data Type Duplicate1/3
  FixPt Switch/1 -> FixPt Data Type Duplicate1/1, Y/1
